simulink model "DPSOPMSM"  (R2013a)
settings: Solver=ode45  StartTime=0.0  StopTime=simtime  FixedStep=1e-3  MaxStep=1e-5  RelTol=1e-3
values from neighbouring files (symbols this model uses):
  fdelay0_1 = 0    [Mainrunme.m]
  J = [0 -1;1 0]    [LIM.m]    (also in Mainrunme.m = 0.005066)
  KI = k(2)    [Mainrunme.m]
  KP = k(1)    [Mainrunme.m]
  minter0_1 = 0    [Mainrunme.m]
  minter0_2 = 0    [Mainrunme.m]
  minter0_3 = 0    [Mainrunme.m]
  minter0_4 = 0    [Mainrunme.m]
  noise_psd_I = (Imax*noise_level/erf_inverse)^2*Ts    (= 6.65228825069e-06)    [Mainrunme.m]
  pidelay0_1 = 0    [Mainrunme.m]
  pidelay0_2 = 0    [Mainrunme.m]
  pidelay0_3 = 0    [Mainrunme.m]
  pidelay0_4 = 0    [Mainrunme.m]
  rand_seed_1 = round(rand*4294967295)    [Mainrunme.m]
  rand_seed_2 = round(rand*4294967295)    [Mainrunme.m]
  Ts = 1e-4    (= 0.0001)    [Mainrunme.m]
undefined symbols (not defined in the file or in its folder): DiscIntNeverNeededParam
libraries: simulink x3
settings Model: SimulationMode=accelerator  Creator=xpwang  LastModifiedBy=wxp
settings OptimizationCC: ExpressionDepthLimit=2147483647  EfficientMapNaN2IntZero=off
settings HardwareCC: TargetIntDivRoundTo=Zero  TargetEndianess=LittleEndian  TargetHWDeviceType=MATLAB Host  ProdEqTarget=off
settings CodeAppCC: MaxIdLength=128
settings GRTTargetCC: CombineOutputUpdateFcns=off  GRTInterface=on

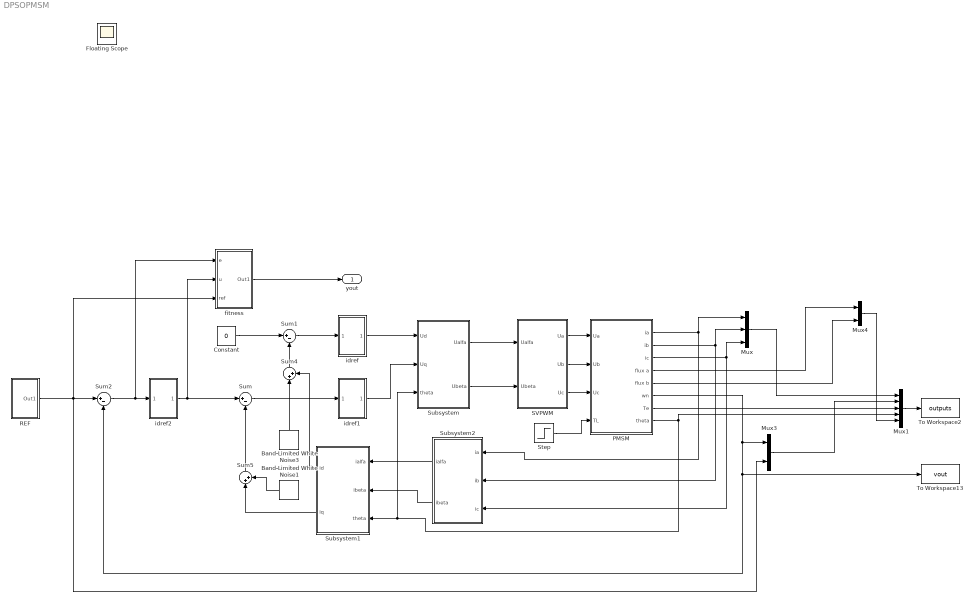
== system DPSOPMSM ==
  Band-Limited White Noise1 : simulink/Sources/Band-Limited White Noise  Cov=[noise_psd_I]  Ts=Ts  seed=[rand_seed_2]
  Band-Limited White Noise3 : simulink/Sources/Band-Limited White Noise  Cov=[noise_psd_I]  Ts=Ts  seed=[rand_seed_1]
  Constant : Constant  Value=0
  Mux : Mux  Inputs=3
  Mux1 : Mux  Inputs=5
  Mux3 : Mux  Inputs=2
  Mux4 : Mux  Inputs=2
  PMSM : Subsystem  mask{Ld=15.57e-3, Lq=15.57e-3, r=1.1, flux_r=0.2667, np=4, J=J, B=0}
      mask prompts: Ld "Stator inductance Ld:"; Lq "Stator inductance Lq:"; r "Stator resistance r:"; flux_r "Flux induced by magnet flux_r:"; np "Number of pole pairs np:"; J "Inertia J:"; B "Friction coefficient B:"
      mask Display:
      | disp('PMSM');
      | port_label('input', 1, '\itU_a', 'texmode', 'on');
      | port_label('input', 2, '\itU_b', 'texmode', 'on');
      | port_label('input', 3, '\itU_c', 'texmode', 'on');
      | port_label('input', 4, '\itTL', 'texmode', 'on');
      | port_label('output', 1, '\iti_a', 'texmode', 'on');
      | port_label('output', 2, '\iti_b', 'texmode', 'on');
      | port_label('output', 3, '\iti_c', 'texmode', 'on');
      | port_label('output', 4, '\itflux a', 'texmode', 'on');
      | port_label('output', 5, '\itflux b', 'texmode', 'on');
      | port_label('output', 6, '\itwn', 'texmode', 'on');
      | port_label('output', 7, '\itTe', 'texmode', 'on');
      | port_label('output', 8, '\ittheta', 'texmode', 'on');
  REF : Subsystem
  SVPWM : Subsystem  mask{Ts=Ts, Udc=350}
      mask prompts: Ts "Period of PWM(Ts):"; Udc "Voltage of DC(Udc):"
      mask Display:
      | disp('SVPWM');
      | port_label('input', 1, '\itU_α', 'texmode', 'on');
      | port_label('input', 2, '\itU_β', 'texmode', 'on');
      | port_label('output', 1, '\itU_a', 'texmode', 'on');
      | port_label('output', 2, '\itU_b', 'texmode', 'on');
      | port_label('output', 3, '\itU_c', 'texmode', 'on');
  Step : Step  Time=0.09  Before=5  After=16  SampleTime=Ts
  Subsystem : Subsystem
      mask Display:
      | disp('dq\n to\n αβ');
      | port_label('input', 1, '\itU_d', 'texmode', 'on');
      | port_label('input', 2, '\itU_q', 'texmode', 'on');
      | port_label('input', 3, '\itθ', 'texmode', 'on');
      | port_label('output', 1, '\itU_α', 'texmode', 'on');
      | port_label('output', 2, '\itU_β', 'texmode', 'on');
  Subsystem1 : Subsystem
      mask Display:
      | disp('αβ\n to\n dq');
      | port_label('input', 1, '\iti_α', 'texmode', 'on');
      | port_label('input', 2, '\iti_β', 'texmode', 'on');
      | port_label('input', 3, '\itθ', 'texmode', 'on');
      | port_label('output', 1, '\iti_d', 'texmode', 'on');
      | port_label('output', 2, '\iti_q', 'texmode', 'on');
  Subsystem2 : Subsystem
      mask Display:
      | disp('abc\n to\n αβ');
      | port_label('input', 1, '\iti_a', 'texmode', 'on');
      | port_label('input', 2, '\iti_b', 'texmode', 'on');
      | port_label('input', 3, '\iti_c', 'texmode', 'on');
      | port_label('output', 1, '\iti_α', 'texmode', 'on');
      | port_label('output', 2, '\iti_β', 'texmode', 'on');
  Sum : Sum  Inputs=|+-
  Sum1 : Sum  Inputs=|+-
  Sum2 : Sum  Inputs=|+-
  Sum4 : Sum  Inputs=|++
  Sum5 : Sum  Inputs=|++
  To Workspace13 : ToWorkspace  VariableName=vout  SampleTime=Ts  SaveFormat=Timeseries
  To Workspace2 : ToWorkspace  VariableName=outputs  SampleTime=Ts  SaveFormat=Timeseries
  fitness : Subsystem
  idref : Subsystem  mask(PI controller){KPd=150, KId=5000, set=[-311, 311]}
      mask prompts: KPd "Propotional(P):"; KId "Intergral(I):"; set "Lower and Upper limit of Output"
      mask init:
      | min=set(1);max=set(2);
      mask Display: disp('PI')
  idref1 : Subsystem  mask(PI controller){KPq=150, KIq=5000, set=[-311, 311]}
      mask prompts: KPq "Propotional(P):"; KIq "Intergral(I):"; set "Lower and Upper limit of Output"
      mask init:
      | min=set(1);max=set(2);
      mask Display: disp('PI')
  idref2 : Subsystem  mask(PI controller){KP=KP, KI=KI, set=[-15, 15]}
      mask prompts: KP "Propotional(P):"; KI "Intergral(I):"; set "Lower and Upper limit of Output"
      mask init:
      | min=set(1);max=set(2);
      mask Display: disp('PI')
  yout : Outport
  Floating Scope : Scope
      settings: Floating=on
  wires:
  Constant/1 -> Sum1/1
  Subsystem/1(Ualfa) -> SVPWM/1(Ualfa)
  Subsystem/2(Ubeta) -> SVPWM/2(Ubeta)
  SVPWM/1(Ua) -> PMSM/1(Ua)
  SVPWM/2(Ub) -> PMSM/2(Ub)
  SVPWM/3(Uc) -> PMSM/3(Uc)
  PMSM/7(Te) -> Mux1/3
  PMSM/5(flux b) -> Mux4/2
  idref2/1(Out1) -> fitness/2(u), Sum/1
  Sum/1 -> idref1/1(In1)
  PMSM/1(ia) -> Mux/1, Subsystem2/1(ia)
  PMSM/2(ib) -> Mux/2, Subsystem2/2(ib)
  PMSM/3(ic) -> Mux/3, Subsystem2/3(ic)
  Subsystem2/1(ialfa) -> Subsystem1/1(ialfa)
  Subsystem2/2(ibeta) -> Subsystem1/2(ibeta)
  Subsystem1/2(iq) -> Sum5/1
  idref1/1(Out1) -> Subsystem/2(Uq)
  Step/1 -> PMSM/4(TL)
  PMSM/8(theta) -> Mux1/4, Subsystem/3(theta), Subsystem1/3(theta)
  Mux3/1 -> Mux1/2
  REF/1(Out1) -> fitness/3(ref), Mux3/2, Sum2/1
  Sum2/1 -> fitness/1(e), idref2/1(In1)
  idref/1(Out1) -> Subsystem/1(Ud)
  Sum1/1 -> idref/1(In1)
  fitness/1(Out1) -> yout/1
  PMSM/4(flux a) -> Mux4/1
  Mux4/1 -> Mux1/5
  PMSM/6(wn) -> Sum2/2, To Workspace13/1, Mux3/1
  Sum5/1 -> Sum/2
  Sum4/1 -> Sum1/2
  Subsystem1/1(id) -> Sum4/2
  Band-Limited White Noise1/1 -> Sum5/2
  Band-Limited White Noise3/1 -> Sum4/1
  Mux1/1 -> To Workspace2/1
  Mux/1 -> Mux1/1

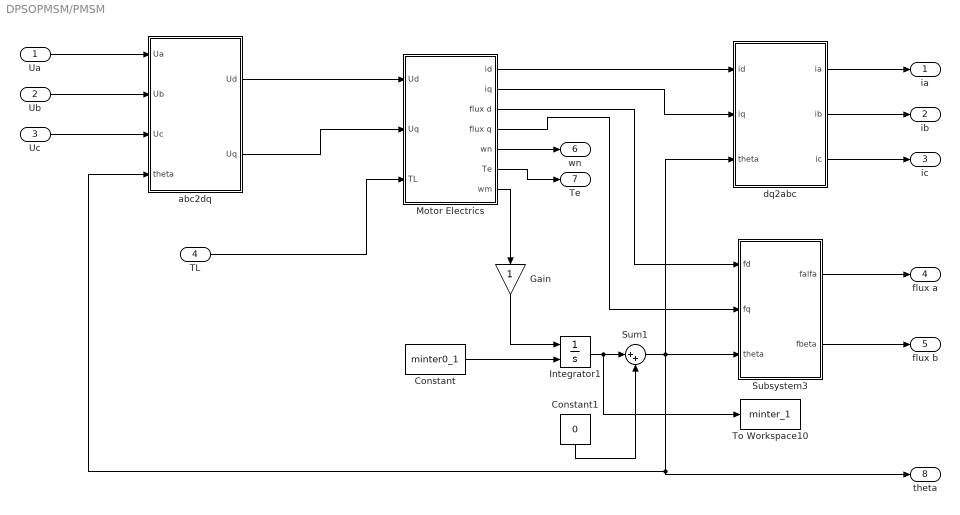
== system DPSOPMSM/PMSM ==
  Ua : Inport
  Ub : Inport  Port=2
  Uc : Inport  Port=3
  TL : Inport  Port=4
  Constant : Constant  Value=minter0_1
  Constant1 : Constant  Value=0
  "Gain " : Gain
  Integrator1 : Integrator  InitialConditionSource=external  InitialCondition=minter0_1
  Motor Electrics : Subsystem
  Subsystem3 : Subsystem
      mask Display:
      | disp('dq\n to\n αβ');
      | port_label('input', 1, '\itflux d', 'texmode', 'on');
      | port_label('input', 2, '\itflux q', 'texmode', 'on');
      | port_label('input', 3, '\itθ', 'texmode', 'on');
      | port_label('output', 1, '\itflux α', 'texmode', 'on');
      | port_label('output', 2, '\itflux β', 'texmode', 'on');
  Sum1 : Sum  Inputs=|++
  To Workspace10 : ToWorkspace  VariableName=minter_1  SampleTime=Ts
      settings: MaxDataPoints=1
  abc2dq : Subsystem
  dq2abc : Subsystem
  ia : Outport
  ib : Outport  Port=2
  ic : Outport  Port=3
  flux a : Outport  Port=4
  flux b : Outport  Port=5
  wn : Outport  Port=6
  Te : Outport  Port=7
  theta : Outport  Port=8
  wires:
  Motor Electrics/3(flux d) -> Subsystem3/1(fd)
  Motor Electrics/4(flux q) -> Subsystem3/2(fq)
  Motor Electrics/5(wn) -> wn/1
  Integrator1/1 -> To Workspace10/1, Sum1/1
  Constant1/1 -> Sum1/2
  Sum1/1 -> dq2abc/3(theta), Subsystem3/3(theta), abc2dq/4(theta), theta/1
  Subsystem3/1(falfa) -> flux a/1
  Subsystem3/2(fbeta) -> flux b/1
  Motor Electrics/6(Te) -> Te/1
  TL/1 -> Motor Electrics/3(TL)
  Motor Electrics/1(id) -> dq2abc/1(id)
  Motor Electrics/2(iq) -> dq2abc/2(iq)
  dq2abc/1(ia) -> ia/1
  dq2abc/2(ib) -> ib/1
  dq2abc/3(ic) -> ic/1
  Ua/1 -> abc2dq/1(Ua)
  Ub/1 -> abc2dq/2(Ub)
  Uc/1 -> abc2dq/3(Uc)
  abc2dq/1(Ud) -> Motor Electrics/1(Ud)
  abc2dq/2(Uq) -> Motor Electrics/2(Uq)
  Motor Electrics/7(wm) -> "Gain "/1
  "Gain "/1 -> Integrator1/1
  Constant/1 -> Integrator1/2

== system DPSOPMSM/REF ==
  Step1 : Step  Time=0.01  After=30  SampleTime=Ts
  Step2 : Step  Time=0.13  After=-30  SampleTime=Ts
  Sum : Sum  Inputs=|++
  To Workspace3 : ToWorkspace  VariableName=v_ref  SampleTime=Ts  SaveFormat=Timeseries
  Zero-Order Hold : ZeroOrderHold  SampleTime=Ts
  Out1 : Outport
  wires:
  Step1/1 -> Sum/1
  Step2/1 -> Sum/2
  Sum/1 -> Zero-Order Hold/1
  Zero-Order Hold/1 -> To Workspace3/1, Out1/1

== system DPSOPMSM/SVPWM ==
  Ualfa : Inport
  Ubeta : Inport  Port=2
  Constant : Constant  Value=Udc
  Constant1 : Constant  Value=Ts
  N1 : Subsystem
  Subsystem : Subsystem
  Subsystem1 : Subsystem
  X.Y.Z : Subsystem
  produce PWM : Subsystem
  Ua : Outport
  Ub : Outport  Port=2
  Uc : Outport  Port=3
  wires:
  Constant1/1 -> X.Y.Z/1(T), Subsystem1/3(T), Subsystem/5(T)
  Constant/1 -> X.Y.Z/4(Udc)
  N1/1(N) -> Subsystem1/4(N), Subsystem/1(N)
  X.Y.Z/1(X) -> Subsystem/2(X)
  X.Y.Z/2(Y) -> Subsystem/3(Y)
  X.Y.Z/3(Z) -> Subsystem/4(Z)
  Subsystem1/1(Tcm1) -> produce PWM/1(Tcm1)
  Subsystem1/2(Tcm2) -> produce PWM/2(Tcm2)
  Subsystem1/3(Tcm3) -> produce PWM/3(Tcm3)
  Ualfa/1 -> X.Y.Z/2(Ualfa), N1/1(Ualfa)
  Subsystem/1(T1) -> Subsystem1/1(T1)
  Subsystem/2(T2) -> Subsystem1/2(T2)
  Ubeta/1 -> N1/2(Ubeta), X.Y.Z/3(Ubeta)
  produce PWM/2(Ub) -> Ub/1
  produce PWM/1(Ua) -> Ua/1
  produce PWM/3(Uc) -> Uc/1

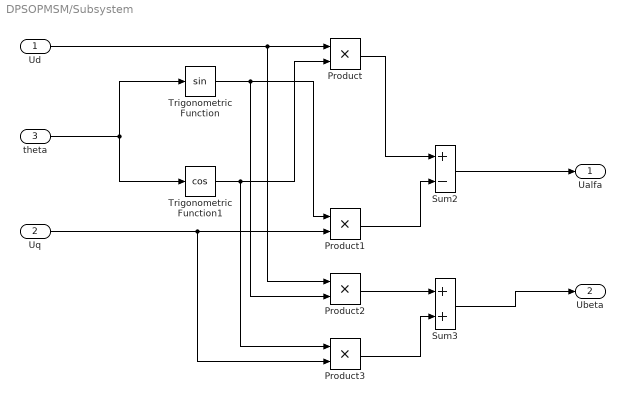
== system DPSOPMSM/Subsystem ==
  Ud : Inport
  Uq : Inport  Port=2
  theta : Inport  Port=3
  Product{,1..3} (4 alike) : Product  RndMeth=Zero
  Sum2 : Sum  Inputs=+-
  Sum3 : Sum
  Trigonometric Function : Trigonometry
  Trigonometric Function1 : Trigonometry  Operator=cos
  Ualfa : Outport
  Ubeta : Outport  Port=2
  wires:
  Product3/1 -> Sum3/2
  Trigonometric Function/1 -> Product2/2, Product1/1
  Product1/1 -> Sum2/2
  Uq/1 -> Product3/2, Product1/2
  Trigonometric Function1/1 -> Product3/1, Product/2
  Ud/1 -> Product2/1, Product/1
  Product/1 -> Sum2/1
  Sum2/1 -> Ualfa/1
  theta/1 -> Trigonometric Function/1, Trigonometric Function1/1
  Product2/1 -> Sum3/1
  Sum3/1 -> Ubeta/1

== system DPSOPMSM/Subsystem1 ==
  ialfa : Inport
  ibeta : Inport  Port=2
  theta : Inport  Port=3
  Product{,1..3} (4 alike) : Product  RndMeth=Zero
  Sum2 : Sum
  Sum3 : Sum  Inputs=+-
  Trigonometric Function : Trigonometry
  Trigonometric Function1 : Trigonometry  Operator=cos
  id : Outport
  iq : Outport  Port=2
  wires:
  Sum3/1 -> iq/1
  Product2/1 -> Sum3/1
  theta/1 -> Trigonometric Function1/1, Trigonometric Function/1
  Sum2/1 -> id/1
  Product/1 -> Sum2/1
  ialfa/1 -> Product3/2, Product/1
  ibeta/1 -> Product2/1, Product1/2
  Product1/1 -> Sum2/2
  Product3/1 -> Sum3/2
  Trigonometric Function1/1 -> Product/2, Product2/2
  Trigonometric Function/1 -> Product3/1, Product1/1

== system DPSOPMSM/Subsystem2 ==
  ia : Inport
  ib : Inport  Port=2
  ic : Inport  Port=3
  Gain : Gain  Gain=1/3
  Gain1 : Gain  Gain=1/sqrt(3)
  Sum2 : Sum  Inputs=+-
  Sum3 : Sum  Inputs=+++
  Sum4 : Sum  Inputs=+-
  ialfa : Outport
  ibeta : Outport  Port=2
  wires:
  Sum2/1 -> Gain1/1
  ic/1 -> Sum3/3, Sum2/2
  Gain1/1 -> ibeta/1
  Sum3/1 -> Gain/1
  Sum4/1 -> ialfa/1
  ib/1 -> Sum3/2, Sum2/1
  Gain/1 -> Sum4/2
  ia/1 -> Sum4/1, Sum3/1

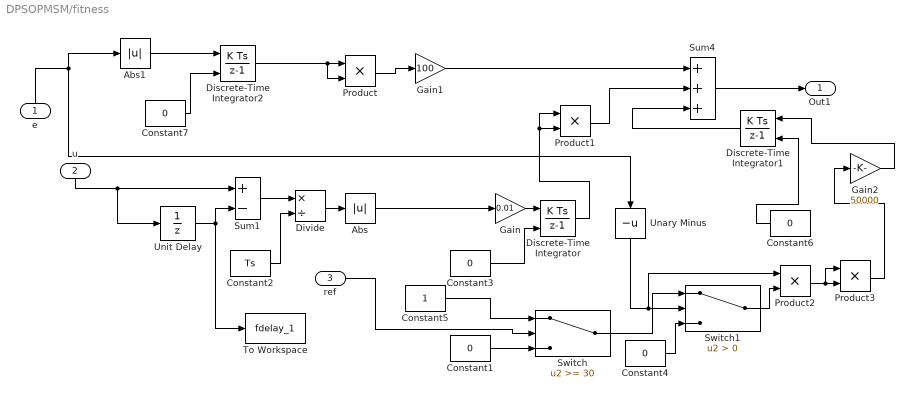
== system DPSOPMSM/fitness ==
  e : Inport
  u : Inport  Port=2
  ref : Inport  Port=3
  Abs : Abs
  Abs1 : Abs
  Constant{1,3..4,6..7} (5 alike) : Constant  Value=0  SampleTime=Ts
  Constant2 : Constant  Value=Ts  SampleTime=Ts
  Constant5 : Constant  SampleTime=Ts
  Discrete-Time Integrator : DiscreteIntegrator  InitialConditionSource=external  SampleTime=Ts  ICPrevOutput=DiscIntNeverNeededParam  ICPrevScaledInput=DiscIntNeverNeededParam
  Discrete-Time Integrator1 : DiscreteIntegrator  InitialConditionSource=external  SampleTime=Ts  ICPrevOutput=DiscIntNeverNeededParam  ICPrevScaledInput=DiscIntNeverNeededParam
  Discrete-Time Integrator2 : DiscreteIntegrator  InitialConditionSource=external  SampleTime=Ts  ICPrevOutput=DiscIntNeverNeededParam  ICPrevScaledInput=DiscIntNeverNeededParam
  Divide : Product  Inputs=*/
  Gain : Gain  Gain=0.01
  Gain1 : Gain  Gain=100
  Gain2 : Gain  Gain=50000
  Product{,1..3} (4 alike) : Product
  Sum1 : Sum  Inputs=+-
  Sum4 : Sum  Inputs=+++
  Switch : Switch  Threshold=30
  Switch1 : Switch  Criteria=u2 > Threshold
  To Workspace : ToWorkspace  VariableName=fdelay_1  SampleTime=-1  SaveFormat=Timeseries
  Unary Minus : UnaryMinus  SampleTime=Ts
  Unit Delay : UnitDelay  InitialCondition=fdelay0_1  SampleTime=-1
  Out1 : Outport
  wires:
  Sum4/1 -> Out1/1
  Gain/1 -> Discrete-Time Integrator/1
  Unit Delay/1 -> To Workspace/1, Sum1/2
  Constant3/1 -> Discrete-Time Integrator/2
  u/1 -> Sum1/1, Unit Delay/1
  Sum1/1 -> Divide/1
  Divide/1 -> Abs/1
  Constant2/1 -> Divide/2
  Gain1/1 -> Sum4/1
  Constant1/1 -> Switch/3
  ref/1 -> Switch/2
  Constant4/1 -> Switch1/3
  Switch/1 -> Switch1/1
  Constant5/1 -> Switch/1
  Switch1/1 -> Product2/2
  Discrete-Time Integrator1/1 -> Sum4/3
  Gain2/1 -> Discrete-Time Integrator1/1
  Constant6/1 -> Discrete-Time Integrator1/2
  Unary Minus/1 -> Product2/1, Switch1/2
  Abs/1 -> Gain/1
  Discrete-Time Integrator2/1 -> Product/2, Product/1
  Product/1 -> Gain1/1
  Discrete-Time Integrator/1 -> Product1/1, Product1/2
  Product3/1 -> Gain2/1
  Product2/1 -> Product3/2, Product3/1
  Product1/1 -> Sum4/2
  e/1 -> Abs1/1, Unary Minus/1
  Constant7/1 -> Discrete-Time Integrator2/2
  Abs1/1 -> Discrete-Time Integrator2/1

== system DPSOPMSM/idref ==
  In1 : Inport
  Add : Sum
  Constant : Constant  Value=Ts
  Inter : Gain  Gain=KId
  Product : Product  RndMeth=Zero
  Propotional : Gain  Gain=KPd
  Saturation : Saturate  UpperLimit=max  LowerLimit=min
  Sum : Sum
  To Workspace5 : ToWorkspace  VariableName=pidelay_2  SampleTime=Ts
      settings: MaxDataPoints=1
  Unit Delay : UnitDelay  InitialCondition=pidelay0_2  SampleTime=-1
  Zero-Order Hold1 : ZeroOrderHold  SampleTime=Ts
  Out1 : Outport
  wires:
  Propotional/1 -> Sum/1
  Product/1 -> Sum/2
  Saturation/1 -> Out1/1
  Add/1 -> Unit Delay/1, Inter/1
  Inter/1 -> Product/1
  Constant/1 -> Product/2
  Sum/1 -> Saturation/1
  In1/1 -> Zero-Order Hold1/1
  Zero-Order Hold1/1 -> Add/1, Propotional/1
  Unit Delay/1 -> To Workspace5/1, Add/2

== system DPSOPMSM/idref1 ==
  In1 : Inport
  Add : Sum
  Constant : Constant  Value=Ts
  Inter : Gain  Gain=KIq
  Product : Product  RndMeth=Zero
  Propotional : Gain  Gain=KPq
  Saturation : Saturate  UpperLimit=max  LowerLimit=min
  Sum : Sum
  To Workspace5 : ToWorkspace  VariableName=pidelay_3  SampleTime=Ts
      settings: MaxDataPoints=1
  Unit Delay : UnitDelay  InitialCondition=pidelay0_3  SampleTime=-1
  Zero-Order Hold1 : ZeroOrderHold  SampleTime=Ts
  Out1 : Outport
  wires:
  Constant/1 -> Product/2
  Inter/1 -> Product/1
  Unit Delay/1 -> To Workspace5/1, Add/2
  Add/1 -> Inter/1, Unit Delay/1
  Saturation/1 -> Out1/1
  Product/1 -> Sum/2
  Propotional/1 -> Sum/1
  Sum/1 -> Saturation/1
  In1/1 -> Zero-Order Hold1/1
  Zero-Order Hold1/1 -> Propotional/1, Add/1

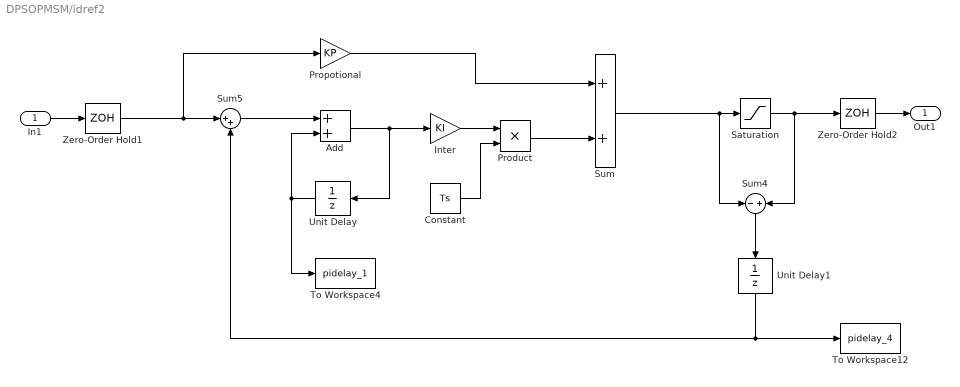
== system DPSOPMSM/idref2 ==
  In1 : Inport
  Add : Sum
  Constant : Constant  Value=Ts
  Inter : Gain  Gain=KI
  Product : Product  RndMeth=Zero
  Propotional : Gain  Gain=KP
  Saturation : Saturate  UpperLimit=max  LowerLimit=min
  Sum : Sum
  Sum4 : Sum  Inputs=-+
  Sum5 : Sum  Inputs=|++
  To Workspace12 : ToWorkspace  VariableName=pidelay_4  SampleTime=Ts
      settings: MaxDataPoints=1
  To Workspace4 : ToWorkspace  VariableName=pidelay_1  SampleTime=Ts
      settings: MaxDataPoints=1
  Unit Delay : UnitDelay  InitialCondition=pidelay0_1  SampleTime=-1
  Unit Delay1 : UnitDelay  InitialCondition=pidelay0_4  SampleTime=Ts
  Zero-Order Hold1 : ZeroOrderHold  SampleTime=Ts
  Zero-Order Hold2 : ZeroOrderHold  SampleTime=Ts
  Out1 : Outport
  wires:
  In1/1 -> Zero-Order Hold1/1
  Propotional/1 -> Sum/1
  Add/1 -> Unit Delay/1, Inter/1
  Unit Delay/1 -> Add/2, To Workspace4/1
  Inter/1 -> Product/1
  Constant/1 -> Product/2
  Saturation/1 -> Sum4/2, Zero-Order Hold2/1
  Unit Delay1/1 -> Sum5/2, To Workspace12/1
  Sum4/1 -> Unit Delay1/1
  Sum5/1 -> Add/1
  Product/1 -> Sum/2
  Zero-Order Hold1/1 -> Propotional/1, Sum5/1
  Sum/1 -> Sum4/1, Saturation/1
  Zero-Order Hold2/1 -> Out1/1

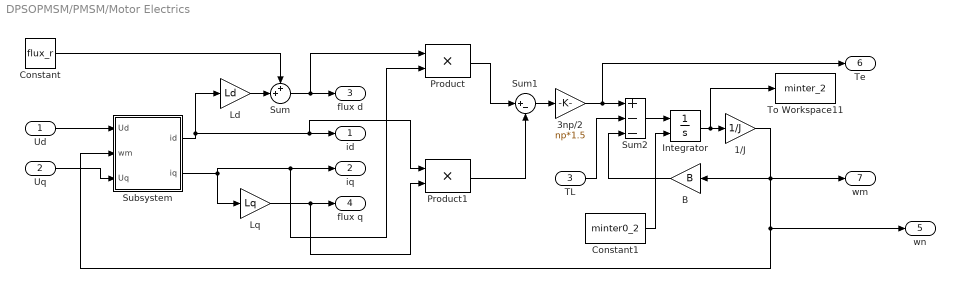
== system DPSOPMSM/PMSM/Motor Electrics ==
  Ud : Inport
  Uq : Inport  Port=2
  TL : Inport  Port=3
  1/J : Gain  Gain=1/J  SaturateOnIntegerOverflow=on  OutDataTypeStr=Inherit: Same as input  ParamDataTypeStr=Inherit: Same as input
  3np/2 : Gain  Gain=np*1.5  SaturateOnIntegerOverflow=on  OutDataTypeStr=Inherit: Same as input  ParamDataTypeStr=Inherit: Same as input
  B : Gain  Gain=B
  Constant : Constant  Value=flux_r
  Constant1 : Constant  Value=minter0_2
  Integrator : Integrator  InitialConditionSource=external  InitialCondition=minter0_2
  Ld : Gain  Gain=Ld  SaturateOnIntegerOverflow=on  OutDataTypeStr=Inherit: Same as input  ParamDataTypeStr=Inherit: Same as input
  Lq : Gain  Gain=Lq  SaturateOnIntegerOverflow=on  OutDataTypeStr=Inherit: Same as input  ParamDataTypeStr=Inherit: Same as input
  Product : Product  SaturateOnIntegerOverflow=on  OutDataTypeStr=Inherit: Same as first input
  Product1 : Product  SaturateOnIntegerOverflow=on  OutDataTypeStr=Inherit: Same as first input
  Subsystem : Subsystem
  Sum : Sum  Inputs=++|  SaturateOnIntegerOverflow=on
  Sum1 : Sum  Inputs=|+-  SaturateOnIntegerOverflow=on
  Sum2 : Sum  Inputs=+--  SaturateOnIntegerOverflow=on
  To Workspace11 : ToWorkspace  VariableName=minter_2  SampleTime=Ts
      settings: MaxDataPoints=1
  id : Outport
  iq : Outport  Port=2
  flux d : Outport  Port=3
  flux q : Outport  Port=4
  wn : Outport  Port=5
  Te : Outport  Port=6
  wm : Outport  Port=7
  wires:
  Integrator/1 -> To Workspace11/1, 1/J/1
  Sum2/1 -> Integrator/1
  TL/1 -> Sum2/2
  3np/2/1 -> Te/1, Sum2/1
  Sum1/1 -> 3np/2/1
  Product1/1 -> Sum1/2
  Product/1 -> Sum1/1
  Lq/1 -> Product1/2, flux q/1
  Sum/1 -> Product/1, flux d/1
  Constant/1 -> Sum/1
  Ld/1 -> Sum/2
  Uq/1 -> Subsystem/3(Uq)
  Subsystem/2(iq) -> Product/2, iq/1, Lq/1
  Ud/1 -> Subsystem/1(Ud)
  Subsystem/1(id) -> Product1/1, id/1, Ld/1
  1/J/1 -> wm/1, Subsystem/2(wm), wn/1, B/1
  B/1 -> Sum2/3
  Constant1/1 -> Integrator/2

== system DPSOPMSM/PMSM/Subsystem3 ==
  fd : Inport
  fq : Inport  Port=2
  theta : Inport  Port=3
  Product{,1..3} (4 alike) : Product  RndMeth=Zero
  Sum2 : Sum  Inputs=+-
  Sum3 : Sum
  Trigonometric Function : Trigonometry
  Trigonometric Function1 : Trigonometry  Operator=cos
  falfa : Outport
  fbeta : Outport  Port=2
  wires:
  Product3/1 -> Sum3/2
  Trigonometric Function/1 -> Product2/2, Product1/1
  Product1/1 -> Sum2/2
  fq/1 -> Product3/2, Product1/2
  Trigonometric Function1/1 -> Product3/1, Product/2
  fd/1 -> Product2/1, Product/1
  Product/1 -> Sum2/1
  Sum2/1 -> falfa/1
  theta/1 -> Trigonometric Function/1, Trigonometric Function1/1
  Product2/1 -> Sum3/1
  Sum3/1 -> fbeta/1

== system DPSOPMSM/PMSM/abc2dq ==
  Ua : Inport
  Ub : Inport  Port=2
  Uc : Inport  Port=3
  theta : Inport  Port=4
  Subsystem1 : Subsystem
      mask Display:
      | disp('αβ\n to\n dq');
      | port_label('input', 1, '\itU_α', 'texmode', 'on');
      | port_label('input', 2, '\itU_β', 'texmode', 'on');
      | port_label('input', 3, '\itθ', 'texmode', 'on');
      | port_label('output', 1, '\itU_d', 'texmode', 'on');
      | port_label('output', 2, '\itU_q', 'texmode', 'on');
  Subsystem2 : Subsystem
      mask Display:
      | disp('abc\n to\n αβ');
      | port_label('input', 1, '\itU_a', 'texmode', 'on');
      | port_label('input', 2, '\itU_b', 'texmode', 'on');
      | port_label('input', 3, '\itU_c', 'texmode', 'on');
      | port_label('output', 1, '\itU_α', 'texmode', 'on');
      | port_label('output', 2, '\itU_β', 'texmode', 'on');
  Ud : Outport
  Uq : Outport  Port=2
  wires:
  Subsystem2/1(Ualfa) -> Subsystem1/1(Ualfa)
  Subsystem2/2(Ubeta) -> Subsystem1/2(Ubeta)
  Subsystem1/1(Ud) -> Ud/1
  Subsystem1/2(Uq) -> Uq/1
  Ua/1 -> Subsystem2/1(Ua)
  Ub/1 -> Subsystem2/2(Ub)
  Uc/1 -> Subsystem2/3(Uc)
  theta/1 -> Subsystem1/3(theta)

== system DPSOPMSM/PMSM/dq2abc ==
  id : Inport
  iq : Inport  Port=2
  theta : Inport  Port=3
  Subsystem4 : Subsystem
      mask Display:
      | disp('αβ\n to\n abc');
      | port_label('input', 1, '\iti_α', 'texmode', 'on');
      | port_label('input', 2, '\iti_β', 'texmode', 'on');
      | port_label('output', 1, '\iti_a', 'texmode', 'on');
      | port_label('output', 2, '\iti_b', 'texmode', 'on');
      | port_label('output', 3, '\iti_c', 'texmode', 'on');
  Subsystem5 : Subsystem
      mask Display:
      | disp('dq\n to\n αβ');
      | port_label('input', 1, '\iti_d', 'texmode', 'on');
      | port_label('input', 2, '\iti_q', 'texmode', 'on');
      | port_label('input', 3, '\itθ', 'texmode', 'on');
      | port_label('output', 1, '\iti_α', 'texmode', 'on');
      | port_label('output', 2, '\iti_β', 'texmode', 'on');
  ia : Outport
  ib : Outport  Port=2
  ic : Outport  Port=3
  wires:
  Subsystem5/2(ibeta) -> Subsystem4/2(ibeta)
  Subsystem5/1(ialfa) -> Subsystem4/1(ialfa)
  id/1 -> Subsystem5/1(id)
  iq/1 -> Subsystem5/2(iq)
  Subsystem4/1(ia) -> ia/1
  Subsystem4/2(ib) -> ib/1
  Subsystem4/3(ic) -> ic/1
  theta/1 -> Subsystem5/3(theta)

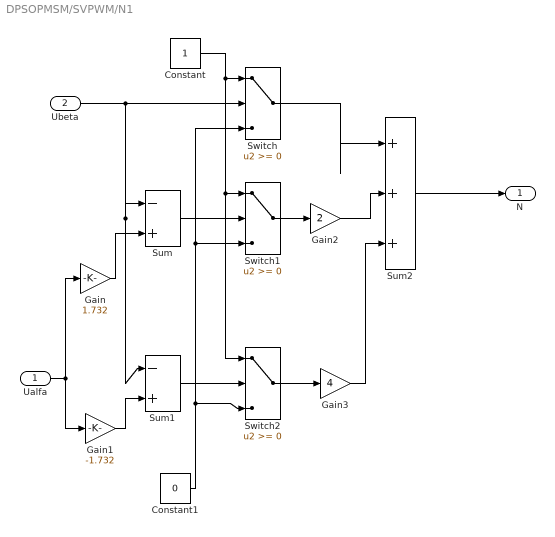
== system DPSOPMSM/SVPWM/N1 ==
  Ualfa : Inport
  Ubeta : Inport  Port=2
  Constant : Constant
  Constant1 : Constant  Value=0
  Gain : Gain  Gain=1.732
  Gain1 : Gain  Gain=-1.732
  Gain2 : Gain  Gain=2
  Gain3 : Gain  Gain=4
  Sum : Sum  Inputs=|-+
  Sum1 : Sum  Inputs=|-+
  Sum2 : Sum  Inputs=|+++
  Switch : Switch  ZeroCross=off
  Switch1 : Switch  ZeroCross=off
  Switch2 : Switch  ZeroCross=off
  N : Outport
  wires:
  Ubeta/1 -> Switch/2, Sum/1, Sum1/1
  Constant/1 -> Switch/1, Switch2/1, Switch1/1
  Ualfa/1 -> Gain1/1, Gain/1
  Gain/1 -> Sum/2
  Sum/1 -> Switch1/2
  Sum1/1 -> Switch2/2
  Gain1/1 -> Sum1/2
  Constant1/1 -> Switch/3, Switch1/3, Switch2/3
  Switch1/1 -> Gain2/1
  Switch2/1 -> Gain3/1
  Gain2/1 -> Sum2/2
  Switch/1 -> Sum2/1
  Gain3/1 -> Sum2/3
  Sum2/1 -> N/1

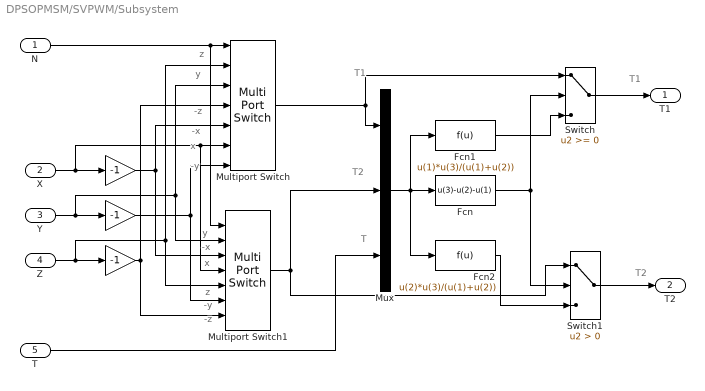
== system DPSOPMSM/SVPWM/Subsystem ==
  note: z
  note: y
  note: -z
  note: -x
  note: x
  note: -y
  note: y
  note: -x
  note: x
  note: z
  note: -y
  note: -z
  note: T1
  note: T2
  note: T
  note: T1
  note: T2
  N : Inport
  X : Inport  Port=2
  Y : Inport  Port=3
  Z : Inport  Port=4
  T : Inport  Port=5
  " " : Gain  Gain=-1
  "  " : Gain  Gain=-1
  "    " : Gain  Gain=-1
  Fcn : Fcn  Expr=u(3)-u(2)-u(1)
  Fcn1 : Fcn  Expr=u(1)*u(3)/(u(1)+u(2))
  Fcn2 : Fcn  Expr=u(2)*u(3)/(u(1)+u(2))
  Multiport Switch : MultiPortSwitch  Inputs=6
  Multiport Switch1 : MultiPortSwitch  Inputs=6
  Mux : Mux  Inputs=3
  Switch : Switch
  Switch1 : Switch  Criteria=u2 > Threshold
  T1 : Outport
  T2 : Outport  Port=2
  wires:
  N/1 -> Multiport Switch1/1, Multiport Switch/1
  X/1 -> Multiport Switch1/4, Multiport Switch/6, " "/1
  Y/1 -> Multiport Switch1/2, Multiport Switch/3, "  "/1
  Z/1 -> Multiport Switch1/5, Multiport Switch/2, "    "/1
  "    "/1 -> Multiport Switch1/7, Multiport Switch/4
  "  "/1 -> Multiport Switch/7, Multiport Switch1/6
  " "/1 -> Multiport Switch/5, Multiport Switch1/3
  Multiport Switch/1 -> Mux/1, Switch/1
  Multiport Switch1/1 -> Switch1/1, Mux/2
  T/1 -> Mux/3
  Mux/1 -> Fcn/1, Fcn1/1, Fcn2/1
  Fcn/1 -> Switch/2, Switch1/2
  Fcn1/1 -> Switch/3
  Fcn2/1 -> Switch1/3
  Switch/1 -> T1/1
  Switch1/1 -> T2/1

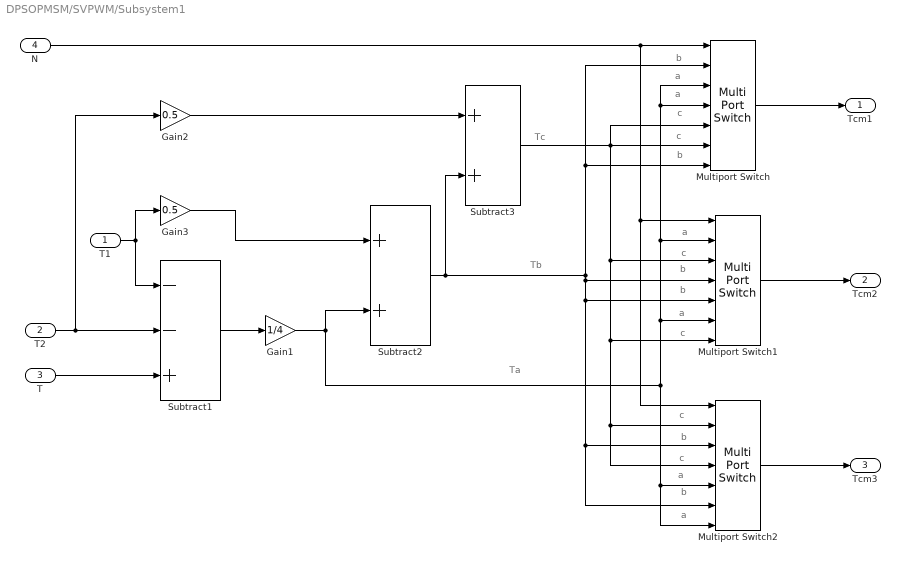
== system DPSOPMSM/SVPWM/Subsystem1 ==
  note: Ta
  note: Tb
  note: Tc
  note: b
  note: a
  note: a
  note: c
  note: c
  note: b
  note: a
  note: c
  note: b
  note: b
  note: a
  note: c
  note: c
  note: b
  note: c
  note: a
  note: b
  note: a
  T1 : Inport
  T2 : Inport  Port=2
  T : Inport  Port=3
  N : Inport  Port=4
  Gain1 : Gain  Gain=1/4
  Gain2 : Gain  Gain=0.5
  Gain3 : Gain  Gain=0.5
  Multiport Switch : MultiPortSwitch  Inputs=6
  Multiport Switch1 : MultiPortSwitch  Inputs=6
  Multiport Switch2 : MultiPortSwitch  Inputs=6
  Subtract1 : Sum  Inputs=--+
  Subtract2 : Sum
  Subtract3 : Sum
  Tcm1 : Outport
  Tcm2 : Outport  Port=2
  Tcm3 : Outport  Port=3
  wires:
  T2/1 -> Gain2/1, Subtract1/2
  T/1 -> Subtract1/3
  T1/1 -> Gain3/1, Subtract1/1
  Gain3/1 -> Subtract2/1
  Subtract1/1 -> Gain1/1
  Gain1/1 -> Subtract2/2, Multiport Switch/3, Multiport Switch/4, Multiport Switch1/2, Multiport Switch1/6, Multiport Switch2/5, Multiport Switch2/7
  Subtract2/1 -> Subtract3/2, Multiport Switch/2, Multiport Switch/7, Multiport Switch1/4, Multiport Switch1/5, Multiport Switch2/3, Multiport Switch2/6
  Gain2/1 -> Subtract3/1
  N/1 -> Multiport Switch/1, Multiport Switch2/1, Multiport Switch1/1
  Multiport Switch/1 -> Tcm1/1
  Multiport Switch1/1 -> Tcm2/1
  Multiport Switch2/1 -> Tcm3/1
  Subtract3/1 -> Multiport Switch/5, Multiport Switch/6, Multiport Switch1/3, Multiport Switch1/7, Multiport Switch2/2, Multiport Switch2/4

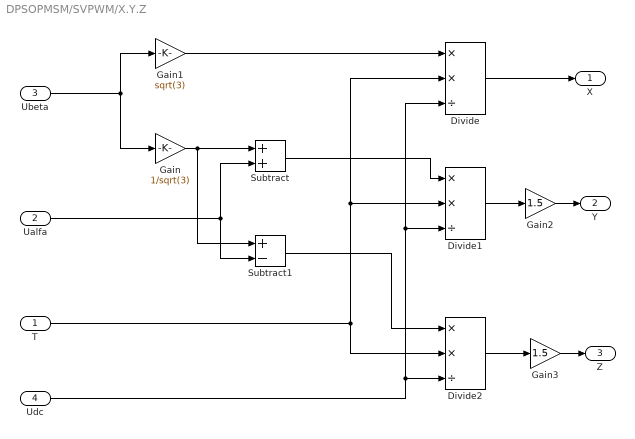
== system DPSOPMSM/SVPWM/X.Y.Z ==
  T : Inport
  Ualfa : Inport  Port=2
  Ubeta : Inport  Port=3
  Udc : Inport  Port=4
  Divide : Product  Inputs=**/
  Divide1 : Product  Inputs=**/
  Divide2 : Product  Inputs=**/
  Gain : Gain  Gain=1/sqrt(3)
  Gain1 : Gain  Gain=sqrt(3)
  Gain2 : Gain  Gain=1.5
  Gain3 : Gain  Gain=1.5
  Subtract : Sum
  Subtract1 : Sum  Inputs=+-
  X : Outport
  Y : Outport  Port=2
  Z : Outport  Port=3
  wires:
  Gain/1 -> Subtract/1, Subtract1/1
  Gain1/1 -> Divide/1
  T/1 -> Divide2/2, Divide1/2, Divide/2
  Udc/1 -> Divide2/3, Divide1/3, Divide/3
  Ualfa/1 -> Subtract/2, Subtract1/2
  Subtract/1 -> Divide1/1
  Subtract1/1 -> Divide2/1
  Divide/1 -> X/1
  Divide1/1 -> Gain2/1
  Divide2/1 -> Gain3/1
  Gain2/1 -> Y/1
  Gain3/1 -> Z/1
  Ubeta/1 -> Gain1/1, Gain/1

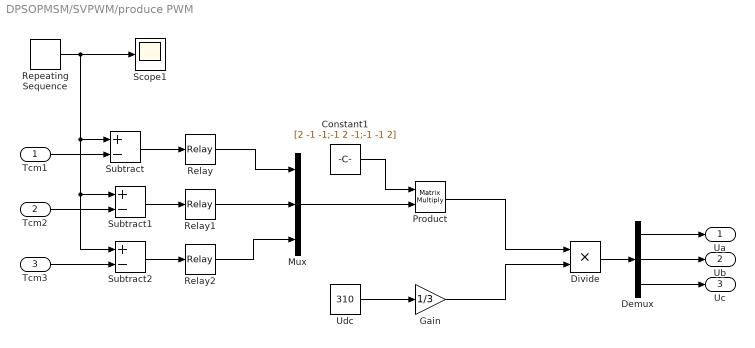
== system DPSOPMSM/SVPWM/produce PWM ==
  Tcm1 : Inport
  Tcm2 : Inport  Port=2
  Tcm3 : Inport  Port=3
  Constant1 : Constant  Value=[2 -1 -1;-1 2 -1;-1 -1 2]
  Demux : Demux  Outputs=3
  Divide : Product  Inputs=**
  Gain : Gain  Gain=1/3
  Mux : Mux  Inputs=3
  Product : Product  Multiplication=Matrix(*)  RndMeth=Zero
  Relay : Relay  OnSwitchValue=2e-10  OffSwitchValue=-2e-10
  Relay1 : Relay  OnSwitchValue=2e-10  OffSwitchValue=-2e-10
  Relay2 : Relay  OnSwitchValue=2e-10  OffSwitchValue=-2e-10
  Repeating Sequence : simulink/Sources/Repeating Sequence  rep_seq_t=[0 Ts/2 Ts]  rep_seq_y=[0 Ts/2 0]
  Scope1 : Scope
      settings: TimeRange=0.3  YMin=0  YMax=2.5e-005  SaveName=ScopeData6
  Subtract : Sum  Inputs=+-
  Subtract1 : Sum  Inputs=+-
  Subtract2 : Sum  Inputs=+-
  Udc : Constant  Value=310
  Ua : Outport
  Ub : Outport  Port=2
  Uc : Outport  Port=3
  wires:
  Subtract/1 -> Relay/1
  Subtract1/1 -> Relay1/1
  Subtract2/1 -> Relay2/1
  Repeating Sequence/1 -> Subtract/1, Subtract2/1, Subtract1/1, Scope1/1
  Tcm1/1 -> Subtract/2
  Tcm2/1 -> Subtract1/2
  Tcm3/1 -> Subtract2/2
  Udc/1 -> Gain/1
  Relay/1 -> Mux/1
  Relay1/1 -> Mux/2
  Relay2/1 -> Mux/3
  Constant1/1 -> Product/1
  Mux/1 -> Product/2
  Product/1 -> Divide/1
  Gain/1 -> Divide/2
  Divide/1 -> Demux/1
  Demux/1 -> Ua/1
  Demux/2 -> Ub/1
  Demux/3 -> Uc/1

== system DPSOPMSM/PMSM/Motor Electrics/Subsystem ==
  Ud : Inport
  wm : Inport  Port=2
  Uq : Inport  Port=3
  Subsystem : Subsystem
  Subsystem1 : Subsystem
  id : Outport
  iq : Outport  Port=2
  wires:
  wm/1 -> Subsystem1/2(wm), Subsystem/2(wm)
  Subsystem/1(id) -> id/1, Subsystem1/1(id)
  Ud/1 -> Subsystem/1(Ud)
  Subsystem1/1(iq) -> iq/1, Subsystem/3(iq)
  Uq/1 -> Subsystem1/3(Uq)

== system DPSOPMSM/PMSM/abc2dq/Subsystem1 ==
  Ualfa : Inport
  Ubeta : Inport  Port=2
  theta : Inport  Port=3
  Product{,1..3} (4 alike) : Product  RndMeth=Zero
  Sum2 : Sum
  Sum3 : Sum  Inputs=+-
  Trigonometric Function : Trigonometry
  Trigonometric Function1 : Trigonometry  Operator=cos
  Ud : Outport
  Uq : Outport  Port=2
  wires:
  Sum3/1 -> Uq/1
  Product2/1 -> Sum3/1
  theta/1 -> Trigonometric Function1/1, Trigonometric Function/1
  Sum2/1 -> Ud/1
  Product/1 -> Sum2/1
  Ualfa/1 -> Product3/2, Product/1
  Ubeta/1 -> Product2/1, Product1/2
  Product1/1 -> Sum2/2
  Product3/1 -> Sum3/2
  Trigonometric Function1/1 -> Product/2, Product2/2
  Trigonometric Function/1 -> Product3/1, Product1/1

== system DPSOPMSM/PMSM/abc2dq/Subsystem2 ==
  Ua : Inport
  Ub : Inport  Port=2
  Uc : Inport  Port=3
  Gain : Gain  Gain=1/3
  Gain1 : Gain  Gain=1/sqrt(3)
  Sum2 : Sum  Inputs=+-
  Sum3 : Sum  Inputs=+++
  Sum4 : Sum  Inputs=+-
  Ualfa : Outport
  Ubeta : Outport  Port=2
  wires:
  Sum2/1 -> Gain1/1
  Uc/1 -> Sum3/3, Sum2/2
  Gain1/1 -> Ubeta/1
  Sum3/1 -> Gain/1
  Sum4/1 -> Ualfa/1
  Ub/1 -> Sum3/2, Sum2/1
  Gain/1 -> Sum4/2
  Ua/1 -> Sum4/1, Sum3/1

== system DPSOPMSM/PMSM/dq2abc/Subsystem4 ==
  ialfa : Inport
  ibeta : Inport  Port=2
  Gain : Gain  Gain=-1/2
  Gain1 : Gain  Gain=sqrt(3)/2
  Sum2 : Sum  Inputs=+-
  Sum4 : Sum
  ia : Outport
  ib : Outport  Port=2
  ic : Outport  Port=3
  wires:
  ialfa/1 -> ia/1, Gain/1
  ibeta/1 -> Gain1/1
  Gain1/1 -> Sum2/2, Sum4/2
  Gain/1 -> Sum2/1, Sum4/1
  Sum4/1 -> ib/1
  Sum2/1 -> ic/1

== system DPSOPMSM/PMSM/dq2abc/Subsystem5 ==
  id : Inport
  iq : Inport  Port=2
  theta : Inport  Port=3
  Product{,1..3} (4 alike) : Product  RndMeth=Zero
  Sum2 : Sum  Inputs=+-
  Sum3 : Sum
  Trigonometric Function : Trigonometry
  Trigonometric Function1 : Trigonometry  Operator=cos
  ialfa : Outport
  ibeta : Outport  Port=2
  wires:
  Sum3/1 -> ibeta/1
  Product2/1 -> Sum3/1
  theta/1 -> Trigonometric Function1/1, Trigonometric Function/1
  Sum2/1 -> ialfa/1
  Product/1 -> Sum2/1
  id/1 -> Product/1, Product2/1
  Trigonometric Function1/1 -> Product/2, Product3/1
  iq/1 -> Product1/2, Product3/2
  Product1/1 -> Sum2/2
  Trigonometric Function/1 -> Product1/1, Product2/2
  Product3/1 -> Sum3/2

== system DPSOPMSM/PMSM/Motor Electrics/Subsystem/Subsystem ==
  Ud : Inport
  wm : Inport  Port=2
  iq : Inport  Port=3
  1/Ld : Gain  Gain=1/Ld  SaturateOnIntegerOverflow=on  OutDataTypeStr=Inherit: Same as input  ParamDataTypeStr=Inherit: Same as input
  Constant2 : Constant  Value=minter0_3
  Integrator : Integrator  InitialConditionSource=external  InitialCondition=minter0_3
  Product : Product  SaturateOnIntegerOverflow=on  OutDataTypeStr=Inherit: Same as first input
  Sum : Sum  Inputs=-++  SaturateOnIntegerOverflow=on
  To Workspace8 : ToWorkspace  VariableName=minter_3  SampleTime=Ts
      settings: MaxDataPoints=1
  np*Lq/Ld : Gain  Gain=np*Lq/Ld  SaturateOnIntegerOverflow=on  OutDataTypeStr=Inherit: Same as input  ParamDataTypeStr=Inherit: Same as input
  r/Ld : Gain  Gain=r/Ld  SaturateOnIntegerOverflow=on  OutDataTypeStr=Inherit: Same as input  ParamDataTypeStr=Inherit: Same as input
  id : Outport
  wires:
  Product/1 -> Sum/3
  np*Lq/Ld/1 -> Product/1
  1/Ld/1 -> Sum/2
  r/Ld/1 -> Sum/1
  Sum/1 -> Integrator/1
  Ud/1 -> 1/Ld/1
  Integrator/1 -> r/Ld/1, id/1, To Workspace8/1
  wm/1 -> Product/2
  iq/1 -> np*Lq/Ld/1
  Constant2/1 -> Integrator/2

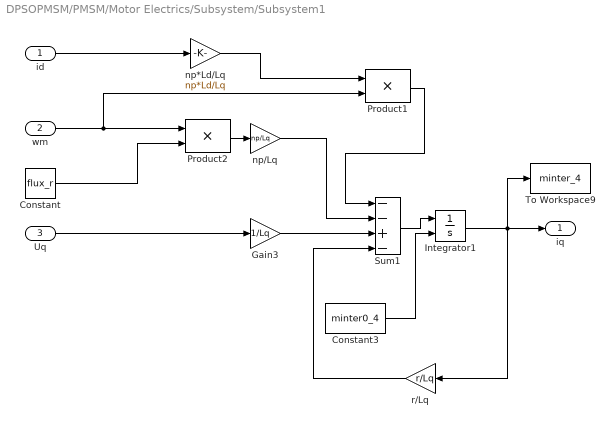
== system DPSOPMSM/PMSM/Motor Electrics/Subsystem/Subsystem1 ==
  id : Inport
  wm : Inport  Port=2
  Uq : Inport  Port=3
  Constant : Constant  Value=flux_r
  Constant3 : Constant  Value=minter0_4
  Gain3 : Gain  Gain=1/Lq  SaturateOnIntegerOverflow=on  OutDataTypeStr=Inherit: Same as input  ParamDataTypeStr=Inherit: Same as input
  Integrator1 : Integrator  InitialConditionSource=external  InitialCondition=minter0_4
  Product1 : Product  SaturateOnIntegerOverflow=on  OutDataTypeStr=Inherit: Same as first input
  Product2 : Product  SaturateOnIntegerOverflow=on  OutDataTypeStr=Inherit: Same as first input
  Sum1 : Sum  Inputs=--+-  SaturateOnIntegerOverflow=on
  To Workspace9 : ToWorkspace  VariableName=minter_4  SampleTime=Ts
      settings: MaxDataPoints=1
  np*Ld/Lq : Gain  Gain=np*Ld/Lq  SaturateOnIntegerOverflow=on  OutDataTypeStr=Inherit: Same as input  ParamDataTypeStr=Inherit: Same as input
  np/Lq : Gain  Gain=np/Lq  SaturateOnIntegerOverflow=on  OutDataTypeStr=Inherit: Same as input  ParamDataTypeStr=Inherit: Same as input
  r/Lq : Gain  Gain=r/Lq  SaturateOnIntegerOverflow=on  OutDataTypeStr=Inherit: Same as input  ParamDataTypeStr=Inherit: Same as input
  iq : Outport
  wires:
  np/Lq/1 -> Sum1/2
  Product2/1 -> np/Lq/1
  Gain3/1 -> Sum1/3
  Constant/1 -> Product2/2
  Integrator1/1 -> r/Lq/1, To Workspace9/1, iq/1
  Product1/1 -> Sum1/1
  Sum1/1 -> Integrator1/1
  Uq/1 -> Gain3/1
  r/Lq/1 -> Sum1/4
  wm/1 -> Product1/2, Product2/1
  np*Ld/Lq/1 -> Product1/1
  id/1 -> np*Ld/Lq/1
  Constant3/1 -> Integrator1/2
